simulink model "MinSegMotor_signal_reconstruction"  (R2024a)
settings: Solver=FixedStepAuto  StartTime=0.0  StopTime=10  FixedStep=1/500  RelTol=1e-3  EnableMultiTasking=on
PostLoadFcn:
  | try,
  | codertarget.arduinobase.registry.setBaudRate(gcs,115200)
  | disp('baud rate set to 115200 for external mode hardware serial')
  | baudrate='set_to_115200'
  | catch
  | disp('baud rate setting not needed in this version')
  | end
undefined symbols (not defined in the file): B_para, f_in, L_t, T_fs, w_k, w_k_IIR
libraries: MinSegLibrary_M2V5 x2
settings Model: SimulationMode=external  ExtModeTrigDuration=2  Creator=Alec  LastModifiedBy=tpjch
settings SolverCC: AlgebraicLoopSolver=TrustRegion  AutoInsertRateTranBlk=on
settings DataIOCC: LimitDataPoints=on  SaveFormat=Array  ReturnWorkspaceOutputs=off
settings OptimizationCC: EnhancedBackFolding=on  PassReuseOutputArgsThreshold=0  ExpressionDepthLimit=2147483647  MaxStackSize=64  OptimizeBlockOrder=speed  DifferentSizesBufferReuse=on  OptimizationCustomize=off
settings DebuggingCC: UnderspecifiedInitializationDetection=Classic  MergeDetectMultiDrivingBlocksExec=none  MultiTaskRateTransMsg=warning  ParameterTunabilityLossMsg=error  UnconnectedInputMsg=warning  UnconnectedOutputMsg=warning  UnconnectedLineMsg=warning  StateNameClashWarn=warning  SFUnexpectedBacktrackingDiag=warning  SFNoUnconditionalDefaultTransitionDiag=warning  SFExecutionAtInitializationDiag=none  ArithmeticOperatorsInVariantConditions=warning
settings HardwareCC: ProdBitPerInt=16  ProdBitPerPointer=16  ProdBitPerSizeT=16  ProdBitPerPtrDiffT=16  ProdLargestAtomicFloat=None  ProdWordSize=8  ProdHWDeviceType=Atmel->AVR  UseEmbeddedCoderFeatures=off  UseSimulinkCoderFeatures=off
settings ModelReferenceCC: PropagateSignalLabelsOutOfModel=off
settings SFSimCC: SimUseLocalCustomCode=off  CustomCodeUndefinedFunction=UseInterfaceOnly
settings RTWCC: Description=Embedded Coder  SystemTargetFile=ert.tlc  HardwareBoard=Arduino Mega 2560  TemplateMakefile=ert_default_tmf  RTWVerbose=off  RTWUseLocalCustomCode=off  Toolchain=Arduino AVR  BuildConfiguration=Faster Runs  GPUComputeCapability=3.5
settings CodeAppCC: ForceParamTrailComments=on  OperatorAnnotations=on  MangleLength=10
settings ERTTargetCC: ERTCustomFileBanners=off  SupportContinuousTime=on  SupportNonInlinedSFcns=on  RemoveResetFunc=off  SupportVariableSizeSignals=on  ModelStepFunctionPrototypeControlCompliant=off  ExtMode=on  ExtModeTransport=3  ExtModeStaticAlloc=on  ExtModeAutomaticAllocSize=off  ExtModeStaticAllocSize=2048  ExtModeMexFile=ext_xcp  ExtModeMexArgs=0 6 115200  ExtModeIntrfLevel=Level2 - Open  ERTSrcFileBannerTemplate=codertarget_code_template.cgt  ERTHdrFileBannerTemplate=codertarget_code_template.cgt  ERTDataSrcFileTemplate=codertarget_code_template.cgt  ERTDataHdrFileTemplate=codertarget_code_template.cgt
settings ConfigComp: CovMetricSettings=dw  CovSaveCumulativeToWorkspaceVar=on  CovSaveSingleToWorkspaceVar=on  CovExternalEMLEnable=off

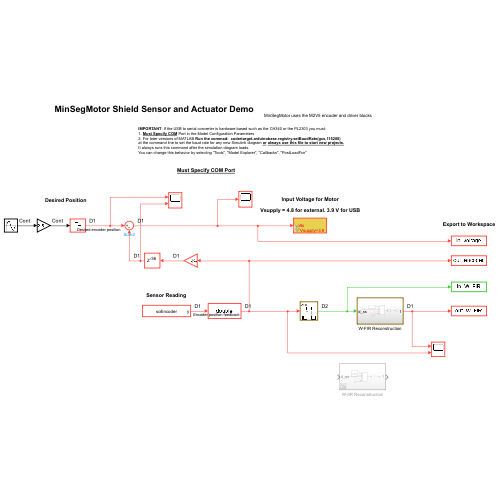
[thumbnail: Simulink's stored preview of the top-level diagram]
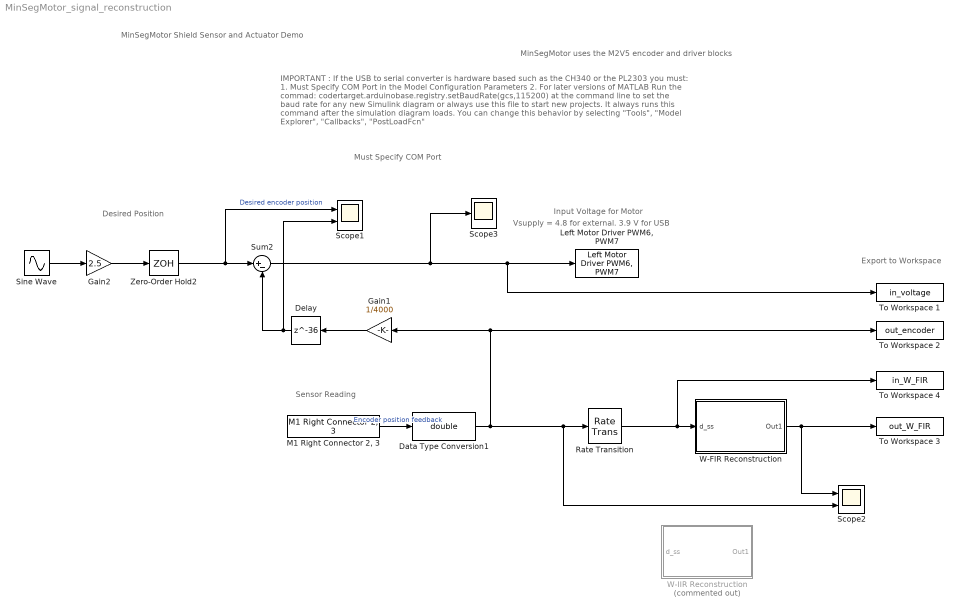
== system MinSegMotor_signal_reconstruction ==
  note: MinSegMotor uses the M2V5 encoder and driver blocks
  note: IMPORTANT : If the USB to serial converter is hardware based such as the CH340 or the PL2303 you must:
      | 1. Must Specify COM Port in the Model Configuration Parameters
      | 2. For later versions of MATLAB Run the commad: codertarget.arduinobase.registry.setBaudRate(gcs,115200)
      | at the command line to set the baud rate for any new Simulink diagram or always use this file to start new projects.
      | It always runs this command after the simulation diagram loads.
      | You can change this behavior by selecting "Tools", "Model Explorer", "Callbacks", "PostLoadFcn"
  note: Must Specify COM Port
  note: Input Voltage for Motor
  note: MinSegMotor Shield Sensor and Actuator Demo
  note: Desired Position
  note: Vsupply = 4.8 for external. 3.9 V for USB
  note: Export to Workspace
  note: Sensor Reading
  Data Type Conversion1 : DataTypeConversion  OutDataTypeStr=double  SaturateOnIntegerOverflow=off  RndMeth=Floor
  Delay : Delay  DelayLength=36
  Gain1 : Gain  Gain=1/4000
  Gain2 : Gain  Gain=2.5
  "Left Motor Driver PWM6, PWM7" : MinSegLibrary_M2V5/Left Motor Driver PWM6, PWM7  Vsupply=3.9  PWMoffset=0
      settings: SourceProductName=M2V5 Library
  "M1 Right Connector 2, 3" : MinSegLibrary_M2V5/M1 Right Connector 2, 3  Encoder=0  PinA=2  PinB=3
      settings: SourceProductName=M2V5 Library
  Rate Transition : RateTransition  OutPortSampleTime=T_ss
  Scope1 : Scope  NumInputPorts=2
  Scope2 : Scope  NumInputPorts=2
  Scope3 : Scope
  Sine Wave : Sin  Frequency=f_in*2*pi  SampleTime=0
  Sum2 : Sum  Inputs=|+-
  To Workspace 1 : ToWorkspace  VariableName=in_voltage  SaveFormat=Structure With Time  SampleTime=-1
      settings: MaxDataPoints=Inf
  To Workspace 2 : ToWorkspace  VariableName=out_encoder  SaveFormat=Structure With Time  SampleTime=-1
      settings: MaxDataPoints=Inf
  To Workspace 3 : ToWorkspace  VariableName=out_W_FIR  SaveFormat=Structure With Time  SampleTime=T_fs
      settings: MaxDataPoints=Inf
  To Workspace 4 : ToWorkspace  VariableName=in_W_FIR  SaveFormat=Structure With Time  SampleTime=-1
      settings: MaxDataPoints=Inf
  W-FIR Reconstruction : Subsystem
  W-IIR Reconstruction : Subsystem  Commented=on
  Zero-Order Hold2 : ZeroOrderHold  SampleTime=T_fs
  wires:
  Rate Transition/1 -> W-FIR Reconstruction/1(d_ss), To Workspace 4/1
  Data Type Conversion1/1 -> Rate Transition/1, Scope2/2, Gain1/1, To Workspace 2/1
  Sum2/1 -> Scope3/1, To Workspace 1/1, "Left Motor Driver PWM6, PWM7"/1
  Sine Wave/1 -> Gain2/1
  Gain2/1 -> Zero-Order Hold2/1
  Zero-Order Hold2/1 -> Scope1/1, Sum2/1  "Desired encoder position"
  "M1 Right Connector 2, 3"/1 -> Data Type Conversion1/1  "Encoder position feedback"
  W-FIR Reconstruction/1(Out1) -> To Workspace 3/1, Scope2/1
  Gain1/1 -> Delay/1
  Delay/1 -> Scope1/2, Sum2/2

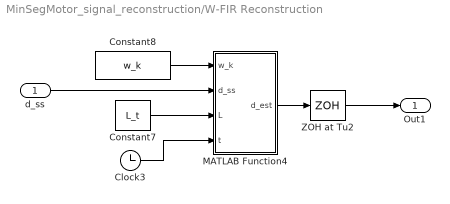
== system MinSegMotor_signal_reconstruction/W-FIR Reconstruction ==
  d_ss : Inport
  Clock3 : Clock
  Constant7 : Constant  Value=L_t
  Constant8 : Constant  Value=w_k
  MATLAB Function4 : MATLAB Function  TreatAsAtomicUnit=on  SystemSampleTime=T_fs
  ZOH at Tu2 : ZeroOrderHold  SampleTime=T_fs
  Out1 : Outport
  wires:
  Constant8/1 -> MATLAB Function4/1(w_k)
  Clock3/1 -> MATLAB Function4/4(t)
  MATLAB Function4/1(d_est) -> ZOH at Tu2/1
  Constant7/1 -> MATLAB Function4/3(L)
  d_ss/1 -> MATLAB Function4/2(d_ss)
  ZOH at Tu2/1 -> Out1/1

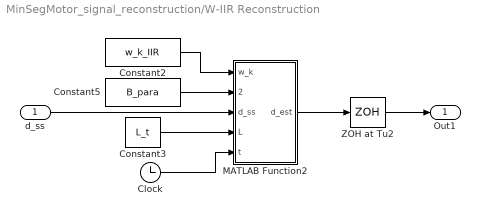
== system MinSegMotor_signal_reconstruction/W-IIR Reconstruction ==
  d_ss : Inport
  Clock : Clock
  Constant2 : Constant  Value=w_k_IIR
  Constant3 : Constant  Value=L_t
  Constant5 : Constant  Value=B_para
  MATLAB Function2 : MATLAB Function  TreatAsAtomicUnit=on  SystemSampleTime=T_fs
  ZOH at Tu2 : ZeroOrderHold  SampleTime=T_fs
  Out1 : Outport
  wires:
  Clock/1 -> MATLAB Function2/5(t)
  Constant2/1 -> MATLAB Function2/1(w_k)
  MATLAB Function2/1(d_est) -> ZOH at Tu2/1
  Constant5/1 -> MATLAB Function2/2(B_para)
  ZOH at Tu2/1 -> Out1/1
  d_ss/1 -> MATLAB Function2/3(d_ss)
  Constant3/1 -> MATLAB Function2/4(L)

== matlab function MinSegMotor_signal_reconstruction/W-FIR Reconstruction/MATLAB Function4 ==
  settings: updateMethod=DISCRETE
  data: w_k input; d_ss input; L input; t input; d_est output
% FIR siganl reconstruction
function d_est = fcn(w_k,d_ss,L,t)
persistent phi n_fs n_ss; % keeps data of variables
n_w = height(w_k); % n_w = 2m elements (index starts at 0,1,...,2m-1)

% assigning initial values
if isempty(phi)
    phi = zeros(1,n_w);
end
if isempty(n_fs)
    n_fs = 0;
end
if isempty(n_ss)
    n_ss = 0;
end

% starts first loop with n_fs = 1 and n_ss = 1
% in MATLAB, d_ss[n_ss] = d_fs[(n_ss-1)*L+1] % for n_ss = 1, ...
% counter for loops performed
n_fs = n_fs+1; % (# of fast samples)
if mod((n_fs-1),L)==0 % update number of slow samples
    n_ss = n_ss + 1; % number of slow samples
end
k = n_fs - (n_ss-1)*L-1; % find the kth intersample point (k = 1,...,L-1)

%% case 1: n_sl < 2*m (not enough data points for FIR)
% case 1 will update phi until there is 2*m slow measured data points
% phi[n] = d_sl[n], phi(1,2m) used to temporarily store the last 2*m ...
% ... measured data points
% 1a: n_sl < 2*m and k=0 means slow and fast measurements match ...
% ... d_sl [n_sl] = d[(n_sl-1)L+1].
% need to update the new set of data points needed to start reconstruction
if (n_ss<n_w) && (k==0)
    for i = 1:(n_w-1)
    phi(n_w-i+1) = phi(n_w-i); % shifts signal data phi(1) -> phi(2)
    end
    phi(1) = d_ss; % current measured data point
    d_est = d_ss; % set d_est = d_ss since the slow and fast align
% when k ~= 0, this is the intersample point, but there is not enough ...
% ... data points, keep this off
elseif (n_ss<n_w) && k~=0 % intersample point estimation
    d_est = 0;
%% case 2: n_sl >= 2m (enough data points for FIR)
% enough data points exist for FIR signal reconstruction
elseif (n_ss>=n_w) && k==0
    for i = 1:(n_w-1)
    phi(n_w-i+1) = phi(n_w-i);
    end
    phi(1) = d_ss;
    d_est = d_ss;
else % final case: n_ss >= n_w && k~=0
    d_est = phi*w_k(:,k); % signal reconstruction step
end

== matlab function MinSegMotor_signal_reconstruction/W-IIR Reconstruction/MATLAB Function2 ==
  settings: updateMethod=DISCRETE
  data: w_k input; B_para input; d_ss input; L input; t input; d_est output
function d_est = fcn(w_k, B_para, d_ss, L, t)
    % Keeps data of variables
    persistent phi n_fs n_ss d_IIR d_IIR_idx;
    n_w = size(w_k, 1); % n_w = 2m elements (index starts at 0,1,...,2m-1)

    % Assigning initial values
    if isempty(phi)
        phi = zeros(1, n_w, 'like', d_ss); % Preallocate phi using the same type as d_ss
    end
    if isempty(n_fs)
        n_fs = 0; % Fast sampling count
    end
    if isempty(n_ss)
        n_ss = 0; % Slow sampling count
    end
    if isempty(d_IIR)
        % Use a smaller buffer size, such as storing only required history
        max_buffer_size = min(2 * n_w * L, 32768); % Limit to 32,768 or less
        d_IIR = zeros(1, max_buffer_size, 'like', d_ss); % Circular buffer
        d_IIR_idx = 1; % Index for circular buffer
    end

    % Increment fast sampling count
    n_fs = n_fs + 1;

    % Update slow sampling count when required
    if mod((n_fs - 1), L) == 0
        n_ss = n_ss + 1; % Number of slow samples
    end

    % Calculate the kth intersample point (k = 1,...,L-1)
    k = n_fs - (n_ss - 1) * L - 1;

    % Case 1: n_ss < n_w (not enough data points for FIR)
    if n_ss < n_w
        if k == 0
            phi = [d_ss, phi(1:end-1)]; % Shift and update phi
            d_est = d_ss; % Fast and slow align
        else
            d_est = 0; % Not enough data for intersample estimation
        end
    % Case 2: n_ss >= n_w (enough data points for FIR)
    elseif n_ss < (n_w + 1)
        if k == 0
            phi = [d_ss, phi(1:end-1)];
            d_est = d_ss;
        else
            d_est = phi * w_k(:, k); % FIR reconstruction
        end
    % Case 3: n_ss >= n_w + 1 (enough data points for IIR)
    else
        if k == 0
            phi = [d_ss, phi(1:end-1)];
            d_est = d_ss;
        else
            % Circular buffer handling
            buffer_start = mod(d_IIR_idx - n_w * L, length(d_IIR)) + 1;
            buffer_indices = buffer_start:L:d_IIR_idx - 1;
            d_est = phi * w_k(:, k) - ...
                flip(d_IIR(buffer_indices)) * B_para(2:end);
        end
    end

    % Update the circular buffer
    d_IIR(d_IIR_idx) = d_est;
    d_IIR_idx = mod(d_IIR_idx, length(d_IIR)) + 1;
end
